simulink model "DataAcquire_debug"  (R2017a)
settings: Solver=FixedStepDiscrete  StartTime=0.0  StopTime=inf  RelTol=1e-3  EnableMultiTasking=on
undefined symbols (not defined in the file or in its folder): T
libraries: simulink x54, stmmbedlib x40
(part 2 of 2)

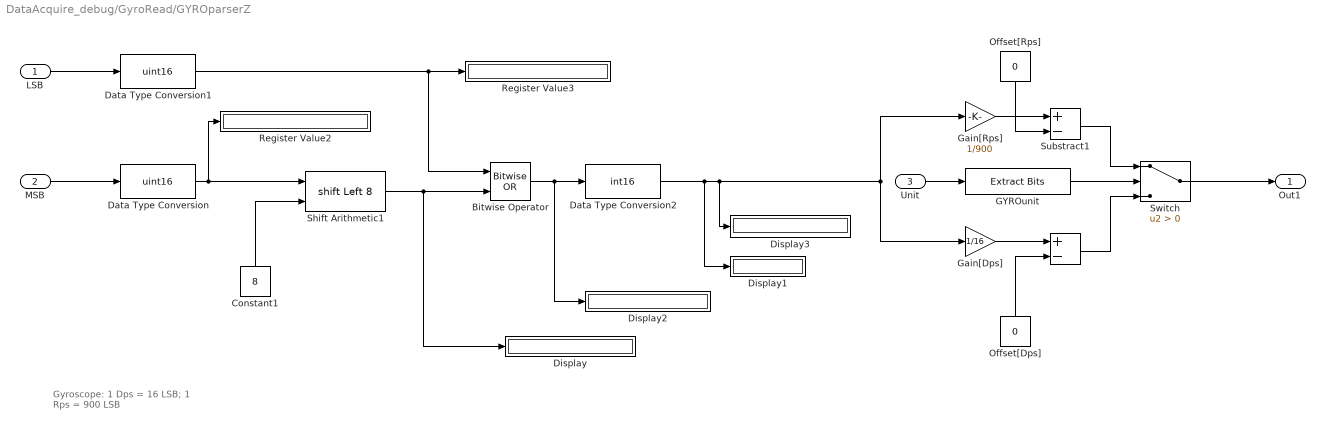
== system DataAcquire_debug/GyroRead/GYROparserZ ==
  note: Gyroscope: 1 Dps = 16 LSB; 1 Rps = 900 LSB
  LSB : Inport
  MSB : Inport  Port=2
  Unit : Inport  Port=3
  " " : Sum  Inputs=+-
  Bitwise Operator : simulink/Logic and Bit Operations/Bitwise Operator  logicop=OR  UseBitMask=off  NumInputPorts=2  BitMask=bin2dec('11011001')  BitMaskRealWorld=Stored Integer
  Constant1 : Constant  Value=8
  Data Type Conversion : DataTypeConversion  OutDataTypeStr=uint16
  Data Type Conversion1 : DataTypeConversion  OutDataTypeStr=uint16
  Data Type Conversion2 : DataTypeConversion  OutDataTypeStr=int16
  Display{,1..3} (4 alike) : Display
      Display settings: Format=binary (Stored Integer)
      Display2 settings: Format=binary (Stored Integer)
      Display3 settings: Format=binary (Stored Integer)
  GYROunit : simulink/Logic and Bit Operations/Extract Bits  bitsToExtract=Range of bits  numBits=8  bitIdxRange=[1 1]  outScalingMode=Preserve fixed-point scaling
      settings: SourceProductName=Simulink
  Gain[Dps] : Gain  Gain=1/16
  Gain[Rps] : Gain  Gain=1/900
  Offset[Dps] : Constant  Value=0
  Offset[Rps] : Constant  Value=0
  Register Value2 : Display
      settings: Format=binary (Stored Integer)
  Register Value3 : Display
      settings: Format=binary (Stored Integer)
  Shift Arithmetic1 : ArithShift  BitShiftNumberSource=Input port  BitShiftNumber=8  BitShiftDirection=Left
      settings: InputPortMap=u0,p1
  Substract1 : Sum  Inputs=+-
  Switch : Switch  Criteria=u2 > Threshold
  Out1 : Outport
  wires:
  Gain[Dps]/1 -> " "/1
  Gain[Rps]/1 -> Substract1/1
  Substract1/1 -> Switch/1
  Offset[Dps]/1 -> " "/2
  Switch/1 -> Out1/1
  " "/1 -> Switch/3
  Offset[Rps]/1 -> Substract1/2
  MSB/1 -> Data Type Conversion/1
  Constant1/1 -> Shift Arithmetic1/2
  Bitwise Operator/1 -> Display2/1, Data Type Conversion2/1
  Shift Arithmetic1/1 -> Display/1, Bitwise Operator/2
  Data Type Conversion1/1 -> Bitwise Operator/1, Register Value3/1
  Data Type Conversion/1 -> Shift Arithmetic1/1, Register Value2/1
  LSB/1 -> Data Type Conversion1/1
  Data Type Conversion2/1 -> Gain[Dps]/1, Gain[Rps]/1, Display3/1, Display1/1
  GYROunit/1 -> Switch/2
  Unit/1 -> GYROunit/1
